simulink model "bus_as_currsource_charging_discharging_final_rearranged"  (R2023a)
settings: Solver=VariableStepAuto  StartTime=0.0  StopTime=10.0  RelTol=1e-3
libraries: spsParallelRLCBranchLib x72, spsCurrentMeasurementLib x27, spsVoltageMeasurementLib x27, spspowerguiLib x25, spsControlledVoltageSourceLib x24, spsVariableResistorLib x24, spsSeriesRLCBranchLib x6, spsMosfetLib x2, sdolib x1, spsControlledCurrentSourceLib x1, spsGroundLib x1
(part 3 of 4)

== system bus_as_currsource_charging_discharging_final_rearranged/Subsystem3 ==
  Clock : Clock
  Controlled Voltage Source : spsControlledVoltageSourceLib/Controlled Voltage Source  Initialize=on  Source_Type=DC  Amplitude=0  Phase=0  Frequency=0  Measurements=None
  Current Measurement : spsCurrentMeasurementLib/Current Measurement  PhasorSimulation=off  OutputType=Complex  PSBequivalent=0
  Delay : Delay  DelayLength=1  InitialCondition=0
  Delay1 : Delay  DelayLength=1  InitialCondition=0
  From1 : From
  From3 : From
  Goto1 : Goto
  Integrator : Integrator
  MATLAB Function : MATLAB Function  TreatAsAtomicUnit=on
  MATLAB Function1 : MATLAB Function  TreatAsAtomicUnit=on
  MATLAB Function2 : MATLAB Function  TreatAsAtomicUnit=on
  Parallel RLC Branch : spsParallelRLCBranchLib/Parallel RLC Branch  LConnTagsString=a  RConnTagsString=__new0  BranchType=RC  Resistance=15.5e-3  Inductance=1e-3  SetiL0=off  InitialCurrent=0  Capacitance=1028.7  Setx0=off  InitialVoltage=0  Measurements=None
  Parallel RLC Branch1 : spsParallelRLCBranchLib/Parallel RLC Branch  LConnTagsString=a  RConnTagsString=__new0  BranchType=RC  Resistance=18.3e-3  Inductance=1e-3  SetiL0=off  InitialCurrent=0  Capacitance=5756.6  Setx0=off  InitialVoltage=0  Measurements=None
  Parallel RLC Branch2 : spsParallelRLCBranchLib/Parallel RLC Branch  LConnTagsString=a  RConnTagsString=__new0  BranchType=R  Resistance=1e9  Inductance=1e-3  SetiL0=off  InitialCurrent=0  Capacitance=5756.6  Setx0=off  InitialVoltage=0  Measurements=None
  Scope2 : Scope
  Scope3 : Scope
  Scope4 : Scope
  Variable Resistor : spsVariableResistorLib/Variable Resistor  Rabsmin=1e-3
      settings: LibrarySourceBlock=sps_lib/Passives/Variable Resistor
  Voltage Measurement1 : spsVoltageMeasurementLib/Voltage Measurement  PhasorSimulation=off  OutputType=Complex  PSBequivalent=0
  XY Graph : Record  FileSettingsInternal="{\"entries\":[{\"content\":{\"excelSettings\":{\"content\":{},\"type\":\"Streamout.ExcelSettings\"}},\"type\":\"Streamout.FileSettingStorage\",\"uuid\":\"c825cdb0-b236-48c7-9482-9a82b7c90d4c\"}],\"packageUris\":[\"http://schema.mathworks.com/mf0/streamout_blocks/R2020a\"],\"version\":\"1.0\"}"  Layout=[1 1]  SignalsInternal="{\"entries\":[{\"content\":{\"signals\":[{\"content\":{\"blockPath\":[\"untitled/Subsystem3/XY Graph\"],\"dimensions\":[1],\"domain\":\"untitled/Subsystem3/XY Graph\",\"lineColor\":\"#fe330a\",\"port\":1,\"signalID\":854,\"signalName\":\"MATLAB Function2\"},\"type\":\"RecordBlkView.Signal\",\"uuid\":\"aa6219c3-15a4-40e1-bdc9-fe25f9f691b4\"},{\"content\":{\"blockPath\":[\"untitled/Subsystem3/XY Graph\"],\"dimensions\":[1],\"domain\":\"untitled/Subsystem3/XY Graph\",\"lineColor\":\"#22b573\",\"port\":2,\"signalID\":857,\"signalName\":\"Voltage Measurement1\"},\"type\":\"RecordBlkView.Signal\",\"uuid\":\"0ce786a2-1d51-4542-a46c-3a9c6b7611eb\"}]},\"type\":\"RecordBlkView.InputSignals\",\"uuid\":\"cce6c00f-2083-4312-89aa-d2be5c477238\"}],\"packageUris\":[\"http://schema.mathworks.com/mf0/streamout_blocks/R2020a\"],\"version\":\"1.0\"}"  VisualizationBindings="{\"xyplotplugin\":{\"info\":[{\"series\":[],\"subplotID\":1}]}}"  CompatibilityTag=XY
  powergui1 : spspowerguiLib/powergui  Priority=1  SimulationMode=Discrete  SampleTime=2e-7  frequency=60  Iterations=50  frequencyindice=0  Pbase=100e6  ErrMax=1e-4  UnitsV=kV  UnitsW=MW  buscounter=0  FunctionMessages=off  echomessages=off  EnableUseOfTLC=off  CurrentSourceSwitches=off  DisableSnubberDevices=off  DisableRonSwitches=off  DisableVfSwitches=off  DisplayEquations=off  AutomaticDiscreteSolvers=off  SolverType=Tustin/Backward Euler (TBE)  Interpol=off  ExternalGateDelay=off  methode=off  Ts=100  x0status=blocks  SPID=on  SwTol=0  HookPort=off  NonlinearTolerance=1e-4  nMaxIteration=100  ContinueOnMaxIteration=off  RestoreLinks=warning  ResistiveCurrentMeasurement=off  Frange=[0:2:500]  Ylog=off  Xlog=on  ShowGrid=off  save=off  variable=ZData  structure=0  ZoomFFT=off  StartTime=0.0  cycles=1  DisplayStyle=1  fundamental=60  FreqAxis=off  MaxFrequency=1000  frequencyindicesteady=1  RmsSteady=1  display=off
  + : PMIOPort  Side=Right
  - : PMIOPort  Port=2  Side=Left
  wires:
  Current Measurement/1 -> Goto1/1
  From3/1 -> Scope3/1
  Voltage Measurement1/1 -> XY Graph/2, Scope2/1
  MATLAB Function2/1(SOC) -> Delay/1, XY Graph/1, Scope4/1
  From1/1 -> Integrator/1
  MATLAB Function/1(y) -> Controlled Voltage Source/1
  MATLAB Function1/1(y) -> Variable Resistor/1
  Integrator/1 -> MATLAB Function2/1(u), MATLAB Function/1(u)
  Clock/1 -> MATLAB Function2/2(time), MATLAB Function/2(time)
  MATLAB Function/2(SOC) -> Delay1/1, MATLAB Function1/1(SOC)
  Delay/1 -> MATLAB Function2/3(SOC1)
  Delay1/1 -> MATLAB Function/3(SOC1)
  connections:
  Variable Resistor/RConn1 -- Parallel RLC Branch/LConn1
  Parallel RLC Branch1/RConn1 -- Parallel RLC Branch2/LConn1 -- +/RConn1 -- Voltage Measurement1/LConn1
  Voltage Measurement1/LConn2 -- Parallel RLC Branch2/RConn1 -- -/RConn1 -- Current Measurement/LConn1
  Controlled Voltage Source/RConn1 -- Variable Resistor/LConn1
  Current Measurement/RConn1 -- Controlled Voltage Source/LConn1
  Parallel RLC Branch/RConn1 -- Parallel RLC Branch1/LConn1

== system bus_as_currsource_charging_discharging_final_rearranged/Subsystem4 ==
  Clock : Clock
  Controlled Voltage Source : spsControlledVoltageSourceLib/Controlled Voltage Source  Initialize=on  Source_Type=DC  Amplitude=0  Phase=0  Frequency=0  Measurements=None
  Current Measurement : spsCurrentMeasurementLib/Current Measurement  PhasorSimulation=off  OutputType=Complex  PSBequivalent=0
  Delay : Delay  DelayLength=1  InitialCondition=0
  Delay1 : Delay  DelayLength=1  InitialCondition=0
  From1 : From
  From3 : From
  Goto1 : Goto
  Integrator : Integrator
  MATLAB Function : MATLAB Function  TreatAsAtomicUnit=on
  MATLAB Function1 : MATLAB Function  TreatAsAtomicUnit=on
  MATLAB Function2 : MATLAB Function  TreatAsAtomicUnit=on
  Parallel RLC Branch : spsParallelRLCBranchLib/Parallel RLC Branch  LConnTagsString=a  RConnTagsString=__new0  BranchType=RC  Resistance=15.5e-3  Inductance=1e-3  SetiL0=off  InitialCurrent=0  Capacitance=1028.7  Setx0=off  InitialVoltage=0  Measurements=None
  Parallel RLC Branch1 : spsParallelRLCBranchLib/Parallel RLC Branch  LConnTagsString=a  RConnTagsString=__new0  BranchType=RC  Resistance=18.3e-3  Inductance=1e-3  SetiL0=off  InitialCurrent=0  Capacitance=5756.6  Setx0=off  InitialVoltage=0  Measurements=None
  Parallel RLC Branch2 : spsParallelRLCBranchLib/Parallel RLC Branch  LConnTagsString=a  RConnTagsString=__new0  BranchType=R  Resistance=1e9  Inductance=1e-3  SetiL0=off  InitialCurrent=0  Capacitance=5756.6  Setx0=off  InitialVoltage=0  Measurements=None
  Scope2 : Scope
  Scope3 : Scope
  Scope4 : Scope
  Variable Resistor : spsVariableResistorLib/Variable Resistor  Rabsmin=1e-3
      settings: LibrarySourceBlock=sps_lib/Passives/Variable Resistor
  Voltage Measurement1 : spsVoltageMeasurementLib/Voltage Measurement  PhasorSimulation=off  OutputType=Complex  PSBequivalent=0
  XY Graph : Record  FileSettingsInternal="{\"entries\":[{\"content\":{\"excelSettings\":{\"content\":{},\"type\":\"Streamout.ExcelSettings\"}},\"type\":\"Streamout.FileSettingStorage\",\"uuid\":\"e9ee8616-40cd-4ee6-9063-a64ba3182807\"}],\"packageUris\":[\"http://schema.mathworks.com/mf0/streamout_blocks/R2020a\"],\"version\":\"1.0\"}"  Layout=[1 1]  SignalsInternal="{\"entries\":[{\"content\":{\"signals\":[{\"content\":{\"blockPath\":[\"untitled/Subsystem4/XY Graph\"],\"dimensions\":[1],\"domain\":\"untitled/Subsystem4/XY Graph\",\"lineColor\":\"#0072bd\",\"port\":1,\"signalID\":862,\"signalName\":\"MATLAB Function2\"},\"type\":\"RecordBlkView.Signal\",\"uuid\":\"dad8bc52-815c-4b8f-9a37-3eeb00578df8\"},{\"content\":{\"blockPath\":[\"untitled/Subsystem4/XY Graph\"],\"dimensions\":[1],\"domain\":\"untitled/Subsystem4/XY Graph\",\"lineColor\":\"#d95319\",\"port\":2,\"signalID\":865,\"signalName\":\"Voltage Measurement1\"},\"type\":\"RecordBlkView.Signal\",\"uuid\":\"40867da1-180e-4687-9423-2f0f6f0d27f3\"}]},\"type\":\"RecordBlkView.InputSignals\",\"uuid\":\"22831997-a808-4c91-ad5b-1ff5947c0370\"}],\"packageUris\":[\"http://schema.mathworks.com/mf0/streamout_blocks/R2020a\"],\"version\":\"1.0\"}"  VisualizationBindings="{\"xyplotplugin\":{\"info\":[{\"series\":[],\"subplotID\":1}]}}"  CompatibilityTag=XY
  powergui1 : spspowerguiLib/powergui  Priority=1  SimulationMode=Discrete  SampleTime=2e-7  frequency=60  Iterations=50  frequencyindice=0  Pbase=100e6  ErrMax=1e-4  UnitsV=kV  UnitsW=MW  buscounter=0  FunctionMessages=off  echomessages=off  EnableUseOfTLC=off  CurrentSourceSwitches=off  DisableSnubberDevices=off  DisableRonSwitches=off  DisableVfSwitches=off  DisplayEquations=off  AutomaticDiscreteSolvers=off  SolverType=Tustin/Backward Euler (TBE)  Interpol=off  ExternalGateDelay=off  methode=off  Ts=100  x0status=blocks  SPID=on  SwTol=0  HookPort=off  NonlinearTolerance=1e-4  nMaxIteration=100  ContinueOnMaxIteration=off  RestoreLinks=warning  ResistiveCurrentMeasurement=off  Frange=[0:2:500]  Ylog=off  Xlog=on  ShowGrid=off  save=off  variable=ZData  structure=0  ZoomFFT=off  StartTime=0.0  cycles=1  DisplayStyle=1  fundamental=60  FreqAxis=off  MaxFrequency=1000  frequencyindicesteady=1  RmsSteady=1  display=off
  + : PMIOPort  Side=Right
  - : PMIOPort  Port=2  Side=Left
  wires:
  Current Measurement/1 -> Goto1/1
  From3/1 -> Scope3/1
  Voltage Measurement1/1 -> XY Graph/2, Scope2/1
  MATLAB Function2/1(SOC) -> Delay/1, XY Graph/1, Scope4/1
  From1/1 -> Integrator/1
  MATLAB Function/1(y) -> Controlled Voltage Source/1
  MATLAB Function1/1(y) -> Variable Resistor/1
  Integrator/1 -> MATLAB Function2/1(u), MATLAB Function/1(u)
  Clock/1 -> MATLAB Function2/2(time), MATLAB Function/2(time)
  MATLAB Function/2(SOC) -> Delay1/1, MATLAB Function1/1(SOC)
  Delay/1 -> MATLAB Function2/3(SOC1)
  Delay1/1 -> MATLAB Function/3(SOC1)
  connections:
  Variable Resistor/RConn1 -- Parallel RLC Branch/LConn1
  Parallel RLC Branch1/RConn1 -- Parallel RLC Branch2/LConn1 -- +/RConn1 -- Voltage Measurement1/LConn1
  Voltage Measurement1/LConn2 -- Parallel RLC Branch2/RConn1 -- -/RConn1 -- Current Measurement/LConn1
  Controlled Voltage Source/RConn1 -- Variable Resistor/LConn1
  Current Measurement/RConn1 -- Controlled Voltage Source/LConn1
  Parallel RLC Branch/RConn1 -- Parallel RLC Branch1/LConn1

== system bus_as_currsource_charging_discharging_final_rearranged/Subsystem5 ==
  Clock : Clock
  Controlled Voltage Source : spsControlledVoltageSourceLib/Controlled Voltage Source  Initialize=on  Source_Type=DC  Amplitude=0  Phase=0  Frequency=0  Measurements=None
  Current Measurement : spsCurrentMeasurementLib/Current Measurement  PhasorSimulation=off  OutputType=Complex  PSBequivalent=0
  Delay : Delay  DelayLength=1  InitialCondition=0
  Delay1 : Delay  DelayLength=1  InitialCondition=0
  From1 : From
  From3 : From
  Goto1 : Goto
  Integrator : Integrator
  MATLAB Function : MATLAB Function  TreatAsAtomicUnit=on
  MATLAB Function1 : MATLAB Function  TreatAsAtomicUnit=on
  MATLAB Function2 : MATLAB Function  TreatAsAtomicUnit=on
  Parallel RLC Branch : spsParallelRLCBranchLib/Parallel RLC Branch  LConnTagsString=a  RConnTagsString=__new0  BranchType=RC  Resistance=15.5e-3  Inductance=1e-3  SetiL0=off  InitialCurrent=0  Capacitance=1028.7  Setx0=off  InitialVoltage=0  Measurements=None
  Parallel RLC Branch1 : spsParallelRLCBranchLib/Parallel RLC Branch  LConnTagsString=a  RConnTagsString=__new0  BranchType=RC  Resistance=18.3e-3  Inductance=1e-3  SetiL0=off  InitialCurrent=0  Capacitance=5756.6  Setx0=off  InitialVoltage=0  Measurements=None
  Parallel RLC Branch2 : spsParallelRLCBranchLib/Parallel RLC Branch  LConnTagsString=a  RConnTagsString=__new0  BranchType=R  Resistance=1e9  Inductance=1e-3  SetiL0=off  InitialCurrent=0  Capacitance=5756.6  Setx0=off  InitialVoltage=0  Measurements=None
  Scope2 : Scope
  Scope3 : Scope
  Scope4 : Scope
  Variable Resistor : spsVariableResistorLib/Variable Resistor  Rabsmin=1e-3
      settings: LibrarySourceBlock=sps_lib/Passives/Variable Resistor
  Voltage Measurement1 : spsVoltageMeasurementLib/Voltage Measurement  PhasorSimulation=off  OutputType=Complex  PSBequivalent=0
  XY Graph : Record  FileSettingsInternal="{\"entries\":[{\"content\":{\"excelSettings\":{\"content\":{},\"type\":\"Streamout.ExcelSettings\"}},\"type\":\"Streamout.FileSettingStorage\",\"uuid\":\"d903b31a-2887-46b6-b9fb-eee4f5b09ecb\"}],\"packageUris\":[\"http://schema.mathworks.com/mf0/streamout_blocks/R2020a\"],\"version\":\"1.0\"}"  Layout=[1 1]  SignalsInternal="{\"entries\":[{\"content\":{\"signals\":[{\"content\":{\"blockPath\":[\"untitled/Subsystem5/XY Graph\"],\"dimensions\":[1],\"domain\":\"untitled/Subsystem5/XY Graph\",\"lineColor\":\"#edb120\",\"port\":1,\"signalID\":870,\"signalName\":\"MATLAB Function2\"},\"type\":\"RecordBlkView.Signal\",\"uuid\":\"92f458b8-da2d-4158-8842-4ef1bbb98961\"},{\"content\":{\"blockPath\":[\"untitled/Subsystem5/XY Graph\"],\"dimensions\":[1],\"domain\":\"untitled/Subsystem5/XY Graph\",\"lineColor\":\"#7e2f8e\",\"port\":2,\"signalID\":873,\"signalName\":\"Voltage Measurement1\"},\"type\":\"RecordBlkView.Signal\",\"uuid\":\"72c3f627-c09a-4660-ae06-75c6e39e2add\"}]},\"type\":\"RecordBlkView.InputSignals\",\"uuid\":\"52288b7e-d80e-4d28-9e0e-4164a3d86710\"}],\"packageUris\":[\"http://schema.mathworks.com/mf0/streamout_blocks/R2020a\"],\"version\":\"1.0\"}"  VisualizationBindings="{\"xyplotplugin\":{\"info\":[{\"series\":[],\"subplotID\":1}]}}"  CompatibilityTag=XY
  powergui1 : spspowerguiLib/powergui  Priority=1  SimulationMode=Discrete  SampleTime=2e-7  frequency=60  Iterations=50  frequencyindice=0  Pbase=100e6  ErrMax=1e-4  UnitsV=kV  UnitsW=MW  buscounter=0  FunctionMessages=off  echomessages=off  EnableUseOfTLC=off  CurrentSourceSwitches=off  DisableSnubberDevices=off  DisableRonSwitches=off  DisableVfSwitches=off  DisplayEquations=off  AutomaticDiscreteSolvers=off  SolverType=Tustin/Backward Euler (TBE)  Interpol=off  ExternalGateDelay=off  methode=off  Ts=100  x0status=blocks  SPID=on  SwTol=0  HookPort=off  NonlinearTolerance=1e-4  nMaxIteration=100  ContinueOnMaxIteration=off  RestoreLinks=warning  ResistiveCurrentMeasurement=off  Frange=[0:2:500]  Ylog=off  Xlog=on  ShowGrid=off  save=off  variable=ZData  structure=0  ZoomFFT=off  StartTime=0.0  cycles=1  DisplayStyle=1  fundamental=60  FreqAxis=off  MaxFrequency=1000  frequencyindicesteady=1  RmsSteady=1  display=off
  + : PMIOPort  Side=Right
  - : PMIOPort  Port=2  Side=Left
  wires:
  Current Measurement/1 -> Goto1/1
  From3/1 -> Scope3/1
  Voltage Measurement1/1 -> XY Graph/2, Scope2/1
  MATLAB Function2/1(SOC) -> Delay/1, XY Graph/1, Scope4/1
  From1/1 -> Integrator/1
  MATLAB Function/1(y) -> Controlled Voltage Source/1
  MATLAB Function1/1(y) -> Variable Resistor/1
  Integrator/1 -> MATLAB Function2/1(u), MATLAB Function/1(u)
  Clock/1 -> MATLAB Function2/2(time), MATLAB Function/2(time)
  MATLAB Function/2(SOC) -> Delay1/1, MATLAB Function1/1(SOC)
  Delay/1 -> MATLAB Function2/3(SOC1)
  Delay1/1 -> MATLAB Function/3(SOC1)
  connections:
  Variable Resistor/RConn1 -- Parallel RLC Branch/LConn1
  Parallel RLC Branch1/RConn1 -- Parallel RLC Branch2/LConn1 -- +/RConn1 -- Voltage Measurement1/LConn1
  Voltage Measurement1/LConn2 -- Parallel RLC Branch2/RConn1 -- -/RConn1 -- Current Measurement/LConn1
  Controlled Voltage Source/RConn1 -- Variable Resistor/LConn1
  Current Measurement/RConn1 -- Controlled Voltage Source/LConn1
  Parallel RLC Branch/RConn1 -- Parallel RLC Branch1/LConn1

== system bus_as_currsource_charging_discharging_final_rearranged/Subsystem6 ==
  Clock : Clock
  Controlled Voltage Source : spsControlledVoltageSourceLib/Controlled Voltage Source  Initialize=on  Source_Type=DC  Amplitude=0  Phase=0  Frequency=0  Measurements=None
  Current Measurement : spsCurrentMeasurementLib/Current Measurement  PhasorSimulation=off  OutputType=Complex  PSBequivalent=0
  Delay : Delay  DelayLength=1  InitialCondition=0
  Delay1 : Delay  DelayLength=1  InitialCondition=0
  From1 : From
  From3 : From
  Goto1 : Goto
  Integrator : Integrator
  MATLAB Function : MATLAB Function  TreatAsAtomicUnit=on
  MATLAB Function1 : MATLAB Function  TreatAsAtomicUnit=on
  MATLAB Function2 : MATLAB Function  TreatAsAtomicUnit=on
  Parallel RLC Branch : spsParallelRLCBranchLib/Parallel RLC Branch  LConnTagsString=a  RConnTagsString=__new0  BranchType=RC  Resistance=15.5e-3  Inductance=1e-3  SetiL0=off  InitialCurrent=0  Capacitance=1028.7  Setx0=off  InitialVoltage=0  Measurements=None
  Parallel RLC Branch1 : spsParallelRLCBranchLib/Parallel RLC Branch  LConnTagsString=a  RConnTagsString=__new0  BranchType=RC  Resistance=18.3e-3  Inductance=1e-3  SetiL0=off  InitialCurrent=0  Capacitance=5756.6  Setx0=off  InitialVoltage=0  Measurements=None
  Parallel RLC Branch2 : spsParallelRLCBranchLib/Parallel RLC Branch  LConnTagsString=a  RConnTagsString=__new0  BranchType=R  Resistance=1e9  Inductance=1e-3  SetiL0=off  InitialCurrent=0  Capacitance=5756.6  Setx0=off  InitialVoltage=0  Measurements=None
  Scope2 : Scope
  Scope3 : Scope
  Scope4 : Scope
  Variable Resistor : spsVariableResistorLib/Variable Resistor  Rabsmin=1e-3
      settings: LibrarySourceBlock=sps_lib/Passives/Variable Resistor
  Voltage Measurement1 : spsVoltageMeasurementLib/Voltage Measurement  PhasorSimulation=off  OutputType=Complex  PSBequivalent=0
  XY Graph : Record  FileSettingsInternal="{\"entries\":[{\"content\":{\"excelSettings\":{\"content\":{},\"type\":\"Streamout.ExcelSettings\"}},\"type\":\"Streamout.FileSettingStorage\",\"uuid\":\"9174c630-a77c-4087-9d74-b4bf6200c048\"}],\"packageUris\":[\"http://schema.mathworks.com/mf0/streamout_blocks/R2020a\"],\"version\":\"1.0\"}"  Layout=[1 1]  SignalsInternal="{\"entries\":[{\"content\":{\"signals\":[{\"content\":{\"blockPath\":[\"untitled/Subsystem6/XY Graph\"],\"dimensions\":[1],\"domain\":\"untitled/Subsystem6/XY Graph\",\"lineColor\":\"#77ac30\",\"port\":1,\"signalID\":878,\"signalName\":\"MATLAB Function2\"},\"type\":\"RecordBlkView.Signal\",\"uuid\":\"0ca10b97-733f-4d6e-a58b-d6abc0f5d709\"},{\"content\":{\"blockPath\":[\"untitled/Subsystem6/XY Graph\"],\"dimensions\":[1],\"domain\":\"untitled/Subsystem6/XY Graph\",\"lineColor\":\"#4dbeee\",\"port\":2,\"signalID\":881,\"signalName\":\"Voltage Measurement1\"},\"type\":\"RecordBlkView.Signal\",\"uuid\":\"186c9fbd-8bc9-44ac-bd9f-d0a4d4dca19a\"}]},\"type\":\"RecordBlkView.InputSignals\",\"uuid\":\"be246018-c51c-40c0-bacb-391947600ef4\"}],\"packageUris\":[\"http://schema.mathworks.com/mf0/streamout_blocks/R2020a\"],\"version\":\"1.0\"}"  VisualizationBindings="{\"xyplotplugin\":{\"info\":[{\"series\":[],\"subplotID\":1}]}}"  CompatibilityTag=XY
  powergui1 : spspowerguiLib/powergui  Priority=1  SimulationMode=Discrete  SampleTime=2e-7  frequency=60  Iterations=50  frequencyindice=0  Pbase=100e6  ErrMax=1e-4  UnitsV=kV  UnitsW=MW  buscounter=0  FunctionMessages=off  echomessages=off  EnableUseOfTLC=off  CurrentSourceSwitches=off  DisableSnubberDevices=off  DisableRonSwitches=off  DisableVfSwitches=off  DisplayEquations=off  AutomaticDiscreteSolvers=off  SolverType=Tustin/Backward Euler (TBE)  Interpol=off  ExternalGateDelay=off  methode=off  Ts=100  x0status=blocks  SPID=on  SwTol=0  HookPort=off  NonlinearTolerance=1e-4  nMaxIteration=100  ContinueOnMaxIteration=off  RestoreLinks=warning  ResistiveCurrentMeasurement=off  Frange=[0:2:500]  Ylog=off  Xlog=on  ShowGrid=off  save=off  variable=ZData  structure=0  ZoomFFT=off  StartTime=0.0  cycles=1  DisplayStyle=1  fundamental=60  FreqAxis=off  MaxFrequency=1000  frequencyindicesteady=1  RmsSteady=1  display=off
  + : PMIOPort  Side=Right
  - : PMIOPort  Port=2  Side=Left
  wires:
  Current Measurement/1 -> Goto1/1
  From3/1 -> Scope3/1
  Voltage Measurement1/1 -> XY Graph/2, Scope2/1
  MATLAB Function2/1(SOC) -> Delay/1, XY Graph/1, Scope4/1
  From1/1 -> Integrator/1
  MATLAB Function/1(y) -> Controlled Voltage Source/1
  MATLAB Function1/1(y) -> Variable Resistor/1
  Integrator/1 -> MATLAB Function2/1(u), MATLAB Function/1(u)
  Clock/1 -> MATLAB Function2/2(time), MATLAB Function/2(time)
  MATLAB Function/2(SOC) -> Delay1/1, MATLAB Function1/1(SOC)
  Delay/1 -> MATLAB Function2/3(SOC1)
  Delay1/1 -> MATLAB Function/3(SOC1)
  connections:
  Variable Resistor/RConn1 -- Parallel RLC Branch/LConn1
  Parallel RLC Branch1/RConn1 -- Parallel RLC Branch2/LConn1 -- +/RConn1 -- Voltage Measurement1/LConn1
  Voltage Measurement1/LConn2 -- Parallel RLC Branch2/RConn1 -- -/RConn1 -- Current Measurement/LConn1
  Controlled Voltage Source/RConn1 -- Variable Resistor/LConn1
  Current Measurement/RConn1 -- Controlled Voltage Source/LConn1
  Parallel RLC Branch/RConn1 -- Parallel RLC Branch1/LConn1

== system bus_as_currsource_charging_discharging_final_rearranged/Subsystem7 ==
  Clock : Clock
  Controlled Voltage Source : spsControlledVoltageSourceLib/Controlled Voltage Source  Initialize=on  Source_Type=DC  Amplitude=0  Phase=0  Frequency=0  Measurements=None
  Current Measurement : spsCurrentMeasurementLib/Current Measurement  PhasorSimulation=off  OutputType=Complex  PSBequivalent=0
  Delay : Delay  DelayLength=1  InitialCondition=0
  Delay1 : Delay  DelayLength=1  InitialCondition=0
  From1 : From
  From3 : From
  Goto1 : Goto
  Integrator : Integrator
  MATLAB Function : MATLAB Function  TreatAsAtomicUnit=on
  MATLAB Function1 : MATLAB Function  TreatAsAtomicUnit=on
  MATLAB Function2 : MATLAB Function  TreatAsAtomicUnit=on
  Parallel RLC Branch : spsParallelRLCBranchLib/Parallel RLC Branch  LConnTagsString=a  RConnTagsString=__new0  BranchType=RC  Resistance=15.5e-3  Inductance=1e-3  SetiL0=off  InitialCurrent=0  Capacitance=1028.7  Setx0=off  InitialVoltage=0  Measurements=None
  Parallel RLC Branch1 : spsParallelRLCBranchLib/Parallel RLC Branch  LConnTagsString=a  RConnTagsString=__new0  BranchType=RC  Resistance=18.3e-3  Inductance=1e-3  SetiL0=off  InitialCurrent=0  Capacitance=5756.6  Setx0=off  InitialVoltage=0  Measurements=None
  Parallel RLC Branch2 : spsParallelRLCBranchLib/Parallel RLC Branch  LConnTagsString=a  RConnTagsString=__new0  BranchType=R  Resistance=1e9  Inductance=1e-3  SetiL0=off  InitialCurrent=0  Capacitance=5756.6  Setx0=off  InitialVoltage=0  Measurements=None
  Scope2 : Scope
  Scope3 : Scope
  Scope4 : Scope
  Variable Resistor : spsVariableResistorLib/Variable Resistor  Rabsmin=1e-3
      settings: LibrarySourceBlock=sps_lib/Passives/Variable Resistor
  Voltage Measurement1 : spsVoltageMeasurementLib/Voltage Measurement  PhasorSimulation=off  OutputType=Complex  PSBequivalent=0
  XY Graph : Record  FileSettingsInternal="{\"entries\":[{\"content\":{\"excelSettings\":{\"content\":{},\"type\":\"Streamout.ExcelSettings\"}},\"type\":\"Streamout.FileSettingStorage\",\"uuid\":\"1f6549a9-b12e-4998-b761-acc27781754e\"}],\"packageUris\":[\"http://schema.mathworks.com/mf0/streamout_blocks/R2020a\"],\"version\":\"1.0\"}"  Layout=[1 1]  SignalsInternal="{\"entries\":[{\"content\":{\"signals\":[{\"content\":{\"blockPath\":[\"untitled/Subsystem7/XY Graph\"],\"dimensions\":[1],\"domain\":\"untitled/Subsystem7/XY Graph\",\"lineColor\":\"#a2142f\",\"port\":1,\"signalID\":886,\"signalName\":\"MATLAB Function2\"},\"type\":\"RecordBlkView.Signal\",\"uuid\":\"c7a6ba5c-6df9-4f2f-bd70-241c1e82a283\"},{\"content\":{\"blockPath\":[\"untitled/Subsystem7/XY Graph\"],\"dimensions\":[1],\"domain\":\"untitled/Subsystem7/XY Graph\",\"lineColor\":\"#139fff\",\"port\":2,\"signalID\":889,\"signalName\":\"Voltage Measurement1\"},\"type\":\"RecordBlkView.Signal\",\"uuid\":\"c35a71e5-140a-452b-8f41-f7cab5fbfd30\"}]},\"type\":\"RecordBlkView.InputSignals\",\"uuid\":\"af273e1b-decb-4944-b23a-6768fa3c0482\"}],\"packageUris\":[\"http://schema.mathworks.com/mf0/streamout_blocks/R2020a\"],\"version\":\"1.0\"}"  VisualizationBindings="{\"xyplotplugin\":{\"info\":[{\"series\":[],\"subplotID\":1}]}}"  CompatibilityTag=XY
  powergui1 : spspowerguiLib/powergui  Priority=1  SimulationMode=Discrete  SampleTime=2e-7  frequency=60  Iterations=50  frequencyindice=0  Pbase=100e6  ErrMax=1e-4  UnitsV=kV  UnitsW=MW  buscounter=0  FunctionMessages=off  echomessages=off  EnableUseOfTLC=off  CurrentSourceSwitches=off  DisableSnubberDevices=off  DisableRonSwitches=off  DisableVfSwitches=off  DisplayEquations=off  AutomaticDiscreteSolvers=off  SolverType=Tustin/Backward Euler (TBE)  Interpol=off  ExternalGateDelay=off  methode=off  Ts=100  x0status=blocks  SPID=on  SwTol=0  HookPort=off  NonlinearTolerance=1e-4  nMaxIteration=100  ContinueOnMaxIteration=off  RestoreLinks=warning  ResistiveCurrentMeasurement=off  Frange=[0:2:500]  Ylog=off  Xlog=on  ShowGrid=off  save=off  variable=ZData  structure=0  ZoomFFT=off  StartTime=0.0  cycles=1  DisplayStyle=1  fundamental=60  FreqAxis=off  MaxFrequency=1000  frequencyindicesteady=1  RmsSteady=1  display=off
  + : PMIOPort  Side=Right
  - : PMIOPort  Port=2  Side=Left
  wires:
  Current Measurement/1 -> Goto1/1
  From3/1 -> Scope3/1
  Voltage Measurement1/1 -> XY Graph/2, Scope2/1
  MATLAB Function2/1(SOC) -> Delay/1, XY Graph/1, Scope4/1
  From1/1 -> Integrator/1
  MATLAB Function/1(y) -> Controlled Voltage Source/1
  MATLAB Function1/1(y) -> Variable Resistor/1
  Integrator/1 -> MATLAB Function2/1(u), MATLAB Function/1(u)
  Clock/1 -> MATLAB Function2/2(time), MATLAB Function/2(time)
  MATLAB Function/2(SOC) -> Delay1/1, MATLAB Function1/1(SOC)
  Delay/1 -> MATLAB Function2/3(SOC1)
  Delay1/1 -> MATLAB Function/3(SOC1)
  connections:
  Variable Resistor/RConn1 -- Parallel RLC Branch/LConn1
  Parallel RLC Branch1/RConn1 -- Parallel RLC Branch2/LConn1 -- +/RConn1 -- Voltage Measurement1/LConn1
  Voltage Measurement1/LConn2 -- Parallel RLC Branch2/RConn1 -- -/RConn1 -- Current Measurement/LConn1
  Controlled Voltage Source/RConn1 -- Variable Resistor/LConn1
  Current Measurement/RConn1 -- Controlled Voltage Source/LConn1
  Parallel RLC Branch/RConn1 -- Parallel RLC Branch1/LConn1

== system bus_as_currsource_charging_discharging_final_rearranged/Subsystem8 ==
  Clock : Clock
  Controlled Voltage Source : spsControlledVoltageSourceLib/Controlled Voltage Source  Initialize=on  Source_Type=DC  Amplitude=0  Phase=0  Frequency=0  Measurements=None
  Current Measurement : spsCurrentMeasurementLib/Current Measurement  PhasorSimulation=off  OutputType=Complex  PSBequivalent=0
  Delay : Delay  DelayLength=1  InitialCondition=0
  Delay1 : Delay  DelayLength=1  InitialCondition=0
  From1 : From
  From3 : From
  Goto1 : Goto
  Integrator : Integrator
  MATLAB Function : MATLAB Function  TreatAsAtomicUnit=on
  MATLAB Function1 : MATLAB Function  TreatAsAtomicUnit=on
  MATLAB Function2 : MATLAB Function  TreatAsAtomicUnit=on
  Parallel RLC Branch : spsParallelRLCBranchLib/Parallel RLC Branch  LConnTagsString=a  RConnTagsString=__new0  BranchType=RC  Resistance=15.5e-3  Inductance=1e-3  SetiL0=off  InitialCurrent=0  Capacitance=1028.7  Setx0=off  InitialVoltage=0  Measurements=None
  Parallel RLC Branch1 : spsParallelRLCBranchLib/Parallel RLC Branch  LConnTagsString=a  RConnTagsString=__new0  BranchType=RC  Resistance=18.3e-3  Inductance=1e-3  SetiL0=off  InitialCurrent=0  Capacitance=5756.6  Setx0=off  InitialVoltage=0  Measurements=None
  Parallel RLC Branch2 : spsParallelRLCBranchLib/Parallel RLC Branch  LConnTagsString=a  RConnTagsString=__new0  BranchType=R  Resistance=1e9  Inductance=1e-3  SetiL0=off  InitialCurrent=0  Capacitance=5756.6  Setx0=off  InitialVoltage=0  Measurements=None
  Scope2 : Scope
  Scope3 : Scope
  Scope4 : Scope
  Variable Resistor : spsVariableResistorLib/Variable Resistor  Rabsmin=1e-3
      settings: LibrarySourceBlock=sps_lib/Passives/Variable Resistor
  Voltage Measurement1 : spsVoltageMeasurementLib/Voltage Measurement  PhasorSimulation=off  OutputType=Complex  PSBequivalent=0
  XY Graph : Record  FileSettingsInternal="{\"entries\":[{\"content\":{\"excelSettings\":{\"content\":{},\"type\":\"Streamout.ExcelSettings\"}},\"type\":\"Streamout.FileSettingStorage\",\"uuid\":\"c27a4e94-2ebe-4191-b8f7-c0309d6a2a71\"}],\"packageUris\":[\"http://schema.mathworks.com/mf0/streamout_blocks/R2020a\"],\"version\":\"1.0\"}"  Layout=[1 1]  SignalsInternal="{\"entries\":[{\"content\":{\"signals\":[{\"content\":{\"blockPath\":[\"untitled/Subsystem8/XY Graph\"],\"dimensions\":[1],\"domain\":\"untitled/Subsystem8/XY Graph\",\"lineColor\":\"#ff6929\",\"port\":1,\"signalID\":894,\"signalName\":\"MATLAB Function2\"},\"type\":\"RecordBlkView.Signal\",\"uuid\":\"b9332481-08d7-48a0-8572-50d15c148681\"},{\"content\":{\"blockPath\":[\"untitled/Subsystem8/XY Graph\"],\"dimensions\":[1],\"domain\":\"untitled/Subsystem8/XY Graph\",\"lineColor\":\"#b746ff\",\"port\":2,\"signalID\":897,\"signalName\":\"Voltage Measurement1\"},\"type\":\"RecordBlkView.Signal\",\"uuid\":\"9a9c2ee4-d070-4202-9ebe-426610b2942d\"}]},\"type\":\"RecordBlkView.InputSignals\",\"uuid\":\"e01ae7b2-176c-4175-96ff-a1ab066f25f0\"}],\"packageUris\":[\"http://schema.mathworks.com/mf0/streamout_blocks/R2020a\"],\"version\":\"1.0\"}"  VisualizationBindings="{\"xyplotplugin\":{\"info\":[{\"series\":[],\"subplotID\":1}]}}"  CompatibilityTag=XY
  powergui1 : spspowerguiLib/powergui  Priority=1  SimulationMode=Discrete  SampleTime=2e-7  frequency=60  Iterations=50  frequencyindice=0  Pbase=100e6  ErrMax=1e-4  UnitsV=kV  UnitsW=MW  buscounter=0  FunctionMessages=off  echomessages=off  EnableUseOfTLC=off  CurrentSourceSwitches=off  DisableSnubberDevices=off  DisableRonSwitches=off  DisableVfSwitches=off  DisplayEquations=off  AutomaticDiscreteSolvers=off  SolverType=Tustin/Backward Euler (TBE)  Interpol=off  ExternalGateDelay=off  methode=off  Ts=100  x0status=blocks  SPID=on  SwTol=0  HookPort=off  NonlinearTolerance=1e-4  nMaxIteration=100  ContinueOnMaxIteration=off  RestoreLinks=warning  ResistiveCurrentMeasurement=off  Frange=[0:2:500]  Ylog=off  Xlog=on  ShowGrid=off  save=off  variable=ZData  structure=0  ZoomFFT=off  StartTime=0.0  cycles=1  DisplayStyle=1  fundamental=60  FreqAxis=off  MaxFrequency=1000  frequencyindicesteady=1  RmsSteady=1  display=off
  + : PMIOPort  Side=Right
  - : PMIOPort  Port=2  Side=Left
  wires:
  Current Measurement/1 -> Goto1/1
  From3/1 -> Scope3/1
  Voltage Measurement1/1 -> XY Graph/2, Scope2/1
  MATLAB Function2/1(SOC) -> Delay/1, XY Graph/1, Scope4/1
  From1/1 -> Integrator/1
  MATLAB Function/1(y) -> Controlled Voltage Source/1
  MATLAB Function1/1(y) -> Variable Resistor/1
  Integrator/1 -> MATLAB Function2/1(u), MATLAB Function/1(u)
  Clock/1 -> MATLAB Function2/2(time), MATLAB Function/2(time)
  MATLAB Function/2(SOC) -> Delay1/1, MATLAB Function1/1(SOC)
  Delay/1 -> MATLAB Function2/3(SOC1)
  Delay1/1 -> MATLAB Function/3(SOC1)
  connections:
  Variable Resistor/RConn1 -- Parallel RLC Branch/LConn1
  Parallel RLC Branch1/RConn1 -- Parallel RLC Branch2/LConn1 -- +/RConn1 -- Voltage Measurement1/LConn1
  Voltage Measurement1/LConn2 -- Parallel RLC Branch2/RConn1 -- -/RConn1 -- Current Measurement/LConn1
  Controlled Voltage Source/RConn1 -- Variable Resistor/LConn1
  Current Measurement/RConn1 -- Controlled Voltage Source/LConn1
  Parallel RLC Branch/RConn1 -- Parallel RLC Branch1/LConn1

== system bus_as_currsource_charging_discharging_final_rearranged/Subsystem9 ==
  Clock : Clock
  Controlled Voltage Source : spsControlledVoltageSourceLib/Controlled Voltage Source  Initialize=on  Source_Type=DC  Amplitude=0  Phase=0  Frequency=0  Measurements=None
  Current Measurement : spsCurrentMeasurementLib/Current Measurement  PhasorSimulation=off  OutputType=Complex  PSBequivalent=0
  Delay : Delay  DelayLength=1  InitialCondition=0
  Delay1 : Delay  DelayLength=1  InitialCondition=0
  From1 : From
  From3 : From
  Goto1 : Goto
  Integrator : Integrator
  MATLAB Function : MATLAB Function  TreatAsAtomicUnit=on
  MATLAB Function1 : MATLAB Function  TreatAsAtomicUnit=on
  MATLAB Function2 : MATLAB Function  TreatAsAtomicUnit=on
  Parallel RLC Branch : spsParallelRLCBranchLib/Parallel RLC Branch  LConnTagsString=a  RConnTagsString=__new0  BranchType=RC  Resistance=15.5e-3  Inductance=1e-3  SetiL0=off  InitialCurrent=0  Capacitance=1028.7  Setx0=off  InitialVoltage=0  Measurements=None
  Parallel RLC Branch1 : spsParallelRLCBranchLib/Parallel RLC Branch  LConnTagsString=a  RConnTagsString=__new0  BranchType=RC  Resistance=18.3e-3  Inductance=1e-3  SetiL0=off  InitialCurrent=0  Capacitance=5756.6  Setx0=off  InitialVoltage=0  Measurements=None
  Parallel RLC Branch2 : spsParallelRLCBranchLib/Parallel RLC Branch  LConnTagsString=a  RConnTagsString=__new0  BranchType=R  Resistance=1e9  Inductance=1e-3  SetiL0=off  InitialCurrent=0  Capacitance=5756.6  Setx0=off  InitialVoltage=0  Measurements=None
  Scope2 : Scope
  Scope3 : Scope
  Scope4 : Scope
  Variable Resistor : spsVariableResistorLib/Variable Resistor  Rabsmin=1e-3
      settings: LibrarySourceBlock=sps_lib/Passives/Variable Resistor
  Voltage Measurement1 : spsVoltageMeasurementLib/Voltage Measurement  PhasorSimulation=off  OutputType=Complex  PSBequivalent=0
  XY Graph : Record  FileSettingsInternal="{\"entries\":[{\"content\":{\"excelSettings\":{\"content\":{},\"type\":\"Streamout.ExcelSettings\"}},\"type\":\"Streamout.FileSettingStorage\",\"uuid\":\"ee199793-1a05-43e1-bde7-51e1bb0f66f6\"}],\"packageUris\":[\"http://schema.mathworks.com/mf0/streamout_blocks/R2020a\"],\"version\":\"1.0\"}"  Layout=[1 1]  SignalsInternal="{\"entries\":[{\"content\":{\"signals\":[{\"content\":{\"blockPath\":[\"untitled/Subsystem9/XY Graph\"],\"dimensions\":[1],\"domain\":\"untitled/Subsystem9/XY Graph\",\"lineColor\":\"#64d413\",\"port\":1,\"signalID\":902,\"signalName\":\"MATLAB Function2\"},\"type\":\"RecordBlkView.Signal\",\"uuid\":\"0c9f0be2-a507-4498-a3f4-26fb21edca4b\"},{\"content\":{\"blockPath\":[\"untitled/Subsystem9/XY Graph\"],\"dimensions\":[1],\"domain\":\"untitled/Subsystem9/XY Graph\",\"lineColor\":\"#ff13a6\",\"port\":2,\"signalID\":905,\"signalName\":\"Voltage Measurement1\"},\"type\":\"RecordBlkView.Signal\",\"uuid\":\"fbc792b1-7c2d-499b-9780-a68ee522e559\"}]},\"type\":\"RecordBlkView.InputSignals\",\"uuid\":\"965ed366-b85e-4589-9108-5f7b37b78915\"}],\"packageUris\":[\"http://schema.mathworks.com/mf0/streamout_blocks/R2020a\"],\"version\":\"1.0\"}"  VisualizationBindings="{\"xyplotplugin\":{\"info\":[{\"series\":[],\"subplotID\":1}]}}"  CompatibilityTag=XY
  powergui1 : spspowerguiLib/powergui  Priority=1  SimulationMode=Discrete  SampleTime=2e-7  frequency=60  Iterations=50  frequencyindice=0  Pbase=100e6  ErrMax=1e-4  UnitsV=kV  UnitsW=MW  buscounter=0  FunctionMessages=off  echomessages=off  EnableUseOfTLC=off  CurrentSourceSwitches=off  DisableSnubberDevices=off  DisableRonSwitches=off  DisableVfSwitches=off  DisplayEquations=off  AutomaticDiscreteSolvers=off  SolverType=Tustin/Backward Euler (TBE)  Interpol=off  ExternalGateDelay=off  methode=off  Ts=100  x0status=blocks  SPID=on  SwTol=0  HookPort=off  NonlinearTolerance=1e-4  nMaxIteration=100  ContinueOnMaxIteration=off  RestoreLinks=warning  ResistiveCurrentMeasurement=off  Frange=[0:2:500]  Ylog=off  Xlog=on  ShowGrid=off  save=off  variable=ZData  structure=0  ZoomFFT=off  StartTime=0.0  cycles=1  DisplayStyle=1  fundamental=60  FreqAxis=off  MaxFrequency=1000  frequencyindicesteady=1  RmsSteady=1  display=off
  + : PMIOPort  Side=Right
  - : PMIOPort  Port=2  Side=Left
  wires:
  Current Measurement/1 -> Goto1/1
  From3/1 -> Scope3/1
  Voltage Measurement1/1 -> XY Graph/2, Scope2/1
  MATLAB Function2/1(SOC) -> Delay/1, XY Graph/1, Scope4/1
  From1/1 -> Integrator/1
  MATLAB Function/1(y) -> Controlled Voltage Source/1
  MATLAB Function1/1(y) -> Variable Resistor/1
  Integrator/1 -> MATLAB Function2/1(u), MATLAB Function/1(u)
  Clock/1 -> MATLAB Function2/2(time), MATLAB Function/2(time)
  MATLAB Function/2(SOC) -> Delay1/1, MATLAB Function1/1(SOC)
  Delay/1 -> MATLAB Function2/3(SOC1)
  Delay1/1 -> MATLAB Function/3(SOC1)
  connections:
  Variable Resistor/RConn1 -- Parallel RLC Branch/LConn1
  Parallel RLC Branch1/RConn1 -- Parallel RLC Branch2/LConn1 -- +/RConn1 -- Voltage Measurement1/LConn1
  Voltage Measurement1/LConn2 -- Parallel RLC Branch2/RConn1 -- -/RConn1 -- Current Measurement/LConn1
  Controlled Voltage Source/RConn1 -- Variable Resistor/LConn1
  Current Measurement/RConn1 -- Controlled Voltage Source/LConn1
  Parallel RLC Branch/RConn1 -- Parallel RLC Branch1/LConn1

== matlab function bus_as_currsource_charging_discharging_final_rearranged/Subsystem1/MATLAB Function ==
  data: u input; y output; time input; SOC output; SOC1 input
function [y,SOC]= fcn(u,time,SOC1)
if time <0.006
    SOC= 60 + 60*u/7920;
else
    SOC=SOC1-SOC1*u/7920;
end
y = 5.56e-5.*SOC.^2+0.001788.*SOC+3.491;

== matlab function bus_as_currsource_charging_discharging_final_rearranged/Subsystem4/MATLAB Function2 ==
  data: u input; SOC output; time input; SOC1 input
function SOC= fcn(u,time,SOC1)
if time <0.006
    SOC= 60 + 60*u/7920;
else
    SOC=SOC1-SOC1*u/7920;
end

== matlab function bus_as_currsource_charging_discharging_final_rearranged/Subsystem5/MATLAB Function ==
  data: u input; y output; time input; SOC output; SOC1 input
function [y,SOC]= fcn(u,time,SOC1)
if time <0.006
    SOC= 60 + 60*u/7920;
else
    SOC=SOC1-SOC1*u/7920;
end
y = 5.56e-5.*SOC.^2+0.001788.*SOC+3.491;

== matlab function bus_as_currsource_charging_discharging_final_rearranged/Subsystem5/MATLAB Function1 ==
  data: SOC input; y output
function y = fcn(SOC)
p1=2.229e-9;
p2=-5.378e-7;
p3=4.791e-5;
p4=-0.001908;
p5=0.08808;
y=p1*SOC^4+p2*SOC^3+p3*SOC^2+p4*SOC+p5;

== matlab function bus_as_currsource_charging_discharging_final_rearranged/Subsystem5/MATLAB Function2 ==
  data: u input; SOC output; time input; SOC1 input
function SOC= fcn(u,time,SOC1)
if time <0.006
    SOC= 60 + 60*u/7920;
else
    SOC=SOC1-SOC1*u/7920;
end

== matlab function bus_as_currsource_charging_discharging_final_rearranged/Subsystem6/MATLAB Function ==
  data: u input; y output; time input; SOC output; SOC1 input
function [y,SOC]= fcn(u,time,SOC1)
if time <0.006
    SOC= 60 + 60*u/7920;
else
    SOC=SOC1-SOC1*u/7920;
end
y = 5.56e-5.*SOC.^2+0.001788.*SOC+3.491;

== matlab function bus_as_currsource_charging_discharging_final_rearranged/Subsystem6/MATLAB Function1 ==
  data: SOC input; y output
function y = fcn(SOC)
p1=2.229e-9;
p2=-5.378e-7;
p3=4.791e-5;
p4=-0.001908;
p5=0.08808;
y=p1*SOC^4+p2*SOC^3+p3*SOC^2+p4*SOC+p5;

== matlab function bus_as_currsource_charging_discharging_final_rearranged/Subsystem6/MATLAB Function2 ==
  data: u input; SOC output; time input; SOC1 input
function SOC= fcn(u,time,SOC1)
if time <0.006
    SOC= 60 + 60*u/7920;
else
    SOC=SOC1-SOC1*u/7920;
end

== matlab function bus_as_currsource_charging_discharging_final_rearranged/Subsystem7/MATLAB Function ==
  data: u input; y output; time input; SOC output; SOC1 input
function [y,SOC]= fcn(u,time,SOC1)
if time <0.006
    SOC= 60 + 60*u/7920;
else
    SOC=SOC1-SOC1*u/7920;
end
y = 5.56e-5.*SOC.^2+0.001788.*SOC+3.491;

== matlab function bus_as_currsource_charging_discharging_final_rearranged/Subsystem7/MATLAB Function1 ==
  data: SOC input; y output
function y = fcn(SOC)
p1=2.229e-9;
p2=-5.378e-7;
p3=4.791e-5;
p4=-0.001908;
p5=0.08808;
y=p1*SOC^4+p2*SOC^3+p3*SOC^2+p4*SOC+p5;

== matlab function bus_as_currsource_charging_discharging_final_rearranged/Subsystem7/MATLAB Function2 ==
  data: u input; SOC output; time input; SOC1 input
function SOC= fcn(u,time,SOC1)
if time <0.006
    SOC= 60 + 60*u/7920;
else
    SOC=SOC1-SOC1*u/7920;
end

== matlab function bus_as_currsource_charging_discharging_final_rearranged/Subsystem8/MATLAB Function ==
  data: u input; y output; time input; SOC output; SOC1 input
function [y,SOC]= fcn(u,time,SOC1)
if time <0.006
    SOC= 60 + 60*u/7920;
else
    SOC=SOC1-SOC1*u/7920;
end
y = 5.56e-5.*SOC.^2+0.001788.*SOC+3.491;

== matlab function bus_as_currsource_charging_discharging_final_rearranged/Subsystem1/MATLAB Function1 ==
  data: SOC input; y output
function y = fcn(SOC)
p1=2.229e-9;
p2=-5.378e-7;
p3=4.791e-5;
p4=-0.001908;
p5=0.08808;
y=p1*SOC^4+p2*SOC^3+p3*SOC^2+p4*SOC+p5;

== matlab function bus_as_currsource_charging_discharging_final_rearranged/Subsystem8/MATLAB Function1 ==
  data: SOC input; y output
function y = fcn(SOC)
p1=2.229e-9;
p2=-5.378e-7;
p3=4.791e-5;
p4=-0.001908;
p5=0.08808;
y=p1*SOC^4+p2*SOC^3+p3*SOC^2+p4*SOC+p5;

== matlab function bus_as_currsource_charging_discharging_final_rearranged/Subsystem8/MATLAB Function2 ==
  data: u input; SOC output; time input; SOC1 input
function SOC= fcn(u,time,SOC1)
if time <0.006
    SOC= 60 + 60*u/7920;
else
    SOC=SOC1-SOC1*u/7920;
end

== matlab function bus_as_currsource_charging_discharging_final_rearranged/Subsystem9/MATLAB Function ==
  data: u input; y output; time input; SOC output; SOC1 input
function [y,SOC]= fcn(u,time,SOC1)
if time <0.006
    SOC= 60 + 60*u/7920;
else
    SOC=SOC1-SOC1*u/7920;
end
y = 5.56e-5.*SOC.^2+0.001788.*SOC+3.491;

== matlab function bus_as_currsource_charging_discharging_final_rearranged/Subsystem9/MATLAB Function1 ==
  data: SOC input; y output
function y = fcn(SOC)
p1=2.229e-9;
p2=-5.378e-7;
p3=4.791e-5;
p4=-0.001908;
p5=0.08808;
y=p1*SOC^4+p2*SOC^3+p3*SOC^2+p4*SOC+p5;

== matlab function bus_as_currsource_charging_discharging_final_rearranged/Subsystem9/MATLAB Function2 ==
  data: u input; SOC output; time input; SOC1 input
function SOC= fcn(u,time,SOC1)
if time <0.006
    SOC= 60 + 60*u/7920;
else
    SOC=SOC1-SOC1*u/7920;
end

== matlab function bus_as_currsource_charging_discharging_final_rearranged/Subsystem10/MATLAB Function ==
  data: u input; y output; time input; SOC output; SOC1 input
function [y,SOC]= fcn(u,time,SOC1)
if time <0.006
    SOC= 60 + 60*u/7920;
else
    SOC=SOC1-SOC1*u/7920;
end
y = 5.56e-5.*SOC.^2+0.001788.*SOC+3.491;

== matlab function bus_as_currsource_charging_discharging_final_rearranged/Subsystem10/MATLAB Function1 ==
  data: SOC input; y output
function y = fcn(SOC)
p1=2.229e-9;
p2=-5.378e-7;
p3=4.791e-5;
p4=-0.001908;
p5=0.08808;
y=p1*SOC^4+p2*SOC^3+p3*SOC^2+p4*SOC+p5;

== matlab function bus_as_currsource_charging_discharging_final_rearranged/Subsystem10/MATLAB Function2 ==
  data: u input; SOC output; time input; SOC1 input
function SOC= fcn(u,time,SOC1)
if time <0.006
    SOC= 60 + 60*u/7920;
else
    SOC=SOC1-SOC1*u/7920;
end

== matlab function bus_as_currsource_charging_discharging_final_rearranged/Subsystem1/MATLAB Function2 ==
  data: u input; SOC output; time input; SOC1 input
function SOC= fcn(u,time,SOC1)
if time <0.006
    SOC= 60 + 60*u/7920;
else
    SOC=SOC1-SOC1*u/7920;
end

== matlab function bus_as_currsource_charging_discharging_final_rearranged/Subsystem11/MATLAB Function ==
  data: u input; y output; time input; SOC output; SOC1 input
function [y,SOC]= fcn(u,time,SOC1)
if time <0.006
    SOC= 60 + 60*u/7920;
else
    SOC=SOC1-SOC1*u/7920;
end
y = 5.56e-5.*SOC.^2+0.001788.*SOC+3.491;

== matlab function bus_as_currsource_charging_discharging_final_rearranged/Subsystem11/MATLAB Function1 ==
  data: SOC input; y output
function y = fcn(SOC)
p1=2.229e-9;
p2=-5.378e-7;
p3=4.791e-5;
p4=-0.001908;
p5=0.08808;
y=p1*SOC^4+p2*SOC^3+p3*SOC^2+p4*SOC+p5;

== matlab function bus_as_currsource_charging_discharging_final_rearranged/Subsystem11/MATLAB Function2 ==
  data: u input; SOC output; time input; SOC1 input
function SOC= fcn(u,time,SOC1)
if time <0.006
    SOC= 60 + 60*u/7920;
else
    SOC=SOC1-SOC1*u/7920;
end

== matlab function bus_as_currsource_charging_discharging_final_rearranged/Subsystem12/MATLAB Function ==
  data: u input; y output; time input; SOC output; SOC1 input
function [y,SOC]= fcn(u,time,SOC1)
if time <0.006
    SOC= 60 + 60*u/7920;
else
    SOC=SOC1-SOC1*u/7920;
end
y = 5.56e-5.*SOC.^2+0.001788.*SOC+3.491;

== matlab function bus_as_currsource_charging_discharging_final_rearranged/Subsystem12/MATLAB Function1 ==
  data: SOC input; y output
function y = fcn(SOC)
p1=2.229e-9;
p2=-5.378e-7;
p3=4.791e-5;
p4=-0.001908;
p5=0.08808;
y=p1*SOC^4+p2*SOC^3+p3*SOC^2+p4*SOC+p5;

== matlab function bus_as_currsource_charging_discharging_final_rearranged/Subsystem12/MATLAB Function2 ==
  data: u input; SOC output; time input; SOC1 input
function SOC= fcn(u,time,SOC1)
if time <0.006
    SOC= 60 + 60*u/7920;
else
    SOC=SOC1-SOC1*u/7920;
end

== matlab function bus_as_currsource_charging_discharging_final_rearranged/Subsystem13/MATLAB Function ==
  data: u input; y output; time input; SOC output; SOC1 input
function [y,SOC]= fcn(u,time,SOC1)
if time <0.006
    SOC= 60 + 60*u/7920;
else
    SOC=SOC1-SOC1*u/7920;
end
y = 5.56e-5.*SOC.^2+0.001788.*SOC+3.491;

== matlab function bus_as_currsource_charging_discharging_final_rearranged/Subsystem13/MATLAB Function1 ==
  data: SOC input; y output
function y = fcn(SOC)
p1=2.229e-9;
p2=-5.378e-7;
p3=4.791e-5;
p4=-0.001908;
p5=0.08808;
y=p1*SOC^4+p2*SOC^3+p3*SOC^2+p4*SOC+p5;

== matlab function bus_as_currsource_charging_discharging_final_rearranged/Subsystem13/MATLAB Function2 ==
  data: u input; SOC output; time input; SOC1 input
function SOC= fcn(u,time,SOC1)
if time <0.006
    SOC= 60 + 60*u/7920;
else
    SOC=SOC1-SOC1*u/7920;
end

== matlab function bus_as_currsource_charging_discharging_final_rearranged/Subsystem14/MATLAB Function ==
  data: u input; y output; time input; SOC output; SOC1 input
function [y,SOC]= fcn(u,time,SOC1)
if time <0.006
    SOC= 60 + 60*u/7920;
else
    SOC=SOC1-SOC1*u/7920;
end
y = 5.56e-5.*SOC.^2+0.001788.*SOC+3.491;

== matlab function bus_as_currsource_charging_discharging_final_rearranged/Subsystem14/MATLAB Function1 ==
  data: SOC input; y output
function y = fcn(SOC)
p1=2.229e-9;
p2=-5.378e-7;
p3=4.791e-5;
p4=-0.001908;
p5=0.08808;
y=p1*SOC^4+p2*SOC^3+p3*SOC^2+p4*SOC+p5;

== matlab function bus_as_currsource_charging_discharging_final_rearranged/Subsystem2/MATLAB Function ==
  data: u input; y output; time input; SOC output; SOC1 input
function [y,SOC]= fcn(u,time,SOC1)
if time <0.006
    SOC= 60 + 60*u/7920;
else
    SOC=SOC1-SOC1*u/7920;
end
y = 5.56e-5.*SOC.^2+0.001788.*SOC+3.491;

== matlab function bus_as_currsource_charging_discharging_final_rearranged/Subsystem14/MATLAB Function2 ==
  data: u input; SOC output; time input; SOC1 input
function SOC= fcn(u,time,SOC1)
if time <0.006
    SOC= 60 + 60*u/7920;
else
    SOC=SOC1-SOC1*u/7920;
end

== matlab function bus_as_currsource_charging_discharging_final_rearranged/Subsystem15/MATLAB Function ==
  data: u input; y output; time input; SOC output; SOC1 input
function [y,SOC]= fcn(u,time,SOC1)
if time <0.006
    SOC= 60 + 60*u/7920;
else
    SOC=SOC1-SOC1*u/7920;
end
y = 5.56e-5.*SOC.^2+0.001788.*SOC+3.491;

== matlab function bus_as_currsource_charging_discharging_final_rearranged/Subsystem15/MATLAB Function1 ==
  data: SOC input; y output
function y = fcn(SOC)
p1=2.229e-9;
p2=-5.378e-7;
p3=4.791e-5;
p4=-0.001908;
p5=0.08808;
y=p1*SOC^4+p2*SOC^3+p3*SOC^2+p4*SOC+p5;

== matlab function bus_as_currsource_charging_discharging_final_rearranged/Subsystem15/MATLAB Function2 ==
  data: u input; SOC output; time input; SOC1 input
function SOC= fcn(u,time,SOC1)
if time <0.006
    SOC= 60 + 60*u/7920;
else
    SOC=SOC1-SOC1*u/7920;
end

== matlab function bus_as_currsource_charging_discharging_final_rearranged/Subsystem16/MATLAB Function ==
  data: u input; y output; time input; SOC output; SOC1 input
function [y,SOC]= fcn(u,time,SOC1)
if time <0.006
    SOC= 60 + 60*u/7920;
else
    SOC=SOC1-SOC1*u/7920;
end
y = 5.56e-5.*SOC.^2+0.001788.*SOC+3.491;

== matlab function bus_as_currsource_charging_discharging_final_rearranged/Subsystem16/MATLAB Function1 ==
  data: SOC input; y output
function y = fcn(SOC)
p1=2.229e-9;
p2=-5.378e-7;
p3=4.791e-5;
p4=-0.001908;
p5=0.08808;
y=p1*SOC^4+p2*SOC^3+p3*SOC^2+p4*SOC+p5;

== matlab function bus_as_currsource_charging_discharging_final_rearranged/Subsystem16/MATLAB Function2 ==
  data: u input; SOC output; time input; SOC1 input
function SOC= fcn(u,time,SOC1)
if time <0.006
    SOC= 60 + 60*u/7920;
else
    SOC=SOC1-SOC1*u/7920;
end

== matlab function bus_as_currsource_charging_discharging_final_rearranged/Subsystem17/MATLAB Function ==
  data: u input; y output; time input; SOC output; SOC1 input
function [y,SOC]= fcn(u,time,SOC1)
if time <0.006
    SOC= 60 + 60*u/7920;
else
    SOC=SOC1-SOC1*u/7920;
end
y = 5.56e-5.*SOC.^2+0.001788.*SOC+3.491;

== matlab function bus_as_currsource_charging_discharging_final_rearranged/Subsystem17/MATLAB Function1 ==
  data: SOC input; y output
function y = fcn(SOC)
p1=2.229e-9;
p2=-5.378e-7;
p3=4.791e-5;
p4=-0.001908;
p5=0.08808;
y=p1*SOC^4+p2*SOC^3+p3*SOC^2+p4*SOC+p5;

== matlab function bus_as_currsource_charging_discharging_final_rearranged/Subsystem17/MATLAB Function2 ==
  data: u input; SOC output; time input; SOC1 input
function SOC= fcn(u,time,SOC1)
if time <0.006
    SOC= 60 + 60*u/7920;
else
    SOC=SOC1-SOC1*u/7920;
end

== matlab function bus_as_currsource_charging_discharging_final_rearranged/Subsystem18/MATLAB Function ==
  data: u input; y output; time input; SOC output; SOC1 input
function [y,SOC]= fcn(u,time,SOC1)
if time <0.006
    SOC= 60 + 60*u/7920;
else
    SOC=SOC1-SOC1*u/7920;
end
y = 5.56e-5.*SOC.^2+0.001788.*SOC+3.491;

== matlab function bus_as_currsource_charging_discharging_final_rearranged/Subsystem2/MATLAB Function1 ==
  data: SOC input; y output
function y = fcn(SOC)
p1=2.229e-9;
p2=-5.378e-7;
p3=4.791e-5;
p4=-0.001908;
p5=0.08808;
y=p1*SOC^4+p2*SOC^3+p3*SOC^2+p4*SOC+p5;
